simulink model "lms"  (R2013a)
settings: Solver=FixedStepDiscrete  StartTime=0.0  StopTime=(samples-1)/fs  RelTol=1e-3
InitFcn:
  | setup;
undefined symbols (not defined in the file or in its folder): fs
libraries: dspadpt3 x1, dspsrcs4 x1
settings Model: Creator=ross  LastModifiedBy=ross
settings DataIOCC: SignalLogging=off
settings OptimizationCC: BlockReduction=off  ConditionallyExecuteInputs=off  InlineParams=on
settings DebuggingCC: AlgebraicLoopMsg=error  Int32ToFloatConvMsg=none
settings HardwareCC: ProdHWDeviceType=ASIC/FPGA->ASIC/FPGA  ProdEqTarget=off

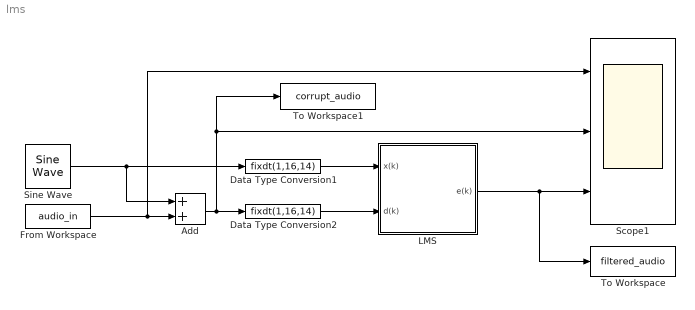
== system lms ==
  Add : Sum
  Data Type Conversion1 : DataTypeConversion  OutDataTypeStr=fixdt(1,16,14)
  Data Type Conversion2 : DataTypeConversion  OutDataTypeStr=fixdt(1,16,14)
  From Workspace : FromWorkspace  VariableName=audio_in  SampleTime=1/fs  Interpolate=off  OutputAfterFinalValue=Holding final value
  LMS : Subsystem
  Scope1 : Scope  NumInputPorts=3
      settings: YMin=-0.5~-1.25~-1  YMax=0.5~1.5~1  MaxDataPoints=samples
  Sine Wave : dspsrcs4/Sine Wave  Amplitude=0.75  Frequency=0.25*fs  Phase=0  SampleMode=Discrete  OutComplex=Real  CompMethod=Table lookup  TableSize=Speed  SampleTime=1/fs  SamplesPerFrame=1  ResetState=Restart at time zero  dataType=Fixed-point  wordLen=16  udDataType=sfix(16)  fracBitsMode=User-defined  numFracBits=14  OutDataTypeStr=fixdt(1,16,14)  LastOutDataTypeStr=fixdt(1,16,14)
  To Workspace : ToWorkspace  VariableName=filtered_audio  SampleTime=-1
  To Workspace1 : ToWorkspace  VariableName=corrupt_audio  SampleTime=-1
  wires:
  Sine Wave/1 -> Add/1, Data Type Conversion1/1
  From Workspace/1 -> Scope1/1, Add/2
  Add/1 -> Data Type Conversion2/1, To Workspace1/1, Scope1/2
  LMS/1(e(k)) -> To Workspace/1, Scope1/3
  Data Type Conversion1/1 -> LMS/1(x(k))
  Data Type Conversion2/1 -> LMS/2(d(k))

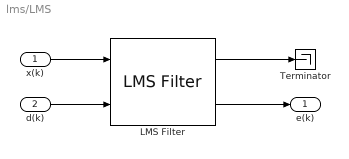
== system lms/LMS ==
  x(k) : Inport
  d(k) : Inport  Port=2
  LMS Filter : dspadpt3/LMS Filter  Algo=LMS  L=16  stepflag=Dialog  mu=0.125  leakage=1.0  ic=0  Adapt=off  resetflag=None  weights=off  secondCoeffMode=User-defined  secondCoeffWordLength=2  secondCoeffFracLength=15  accum2Mode=User-defined  accum2FracLength=20  prodOutput2Mode=User-defined  prodOutput2FracLength=20  prodOutput3Mode=User-defined  prodOutput3FracLength=20  prodOutput4Mode=User-defined  prodOutput4FracLength=20  quotientMode=User-defined  quotientFracLength=20  roundingMode=Convergent  overflowMode=off  addnparflag=off
  Terminator : Terminator
  e(k) : Outport
  wires:
  d(k)/1 -> LMS Filter/2
  x(k)/1 -> LMS Filter/1
  LMS Filter/2 -> e(k)/1
  LMS Filter/1 -> Terminator/1
